simulink model "cwfd"  (R2019b)
settings: Solver=VariableStepAuto  StartTime=0.0  StopTime=10.0  RelTol=1e-3
settings Model: Creator=Blade  LastModifiedBy=Blade

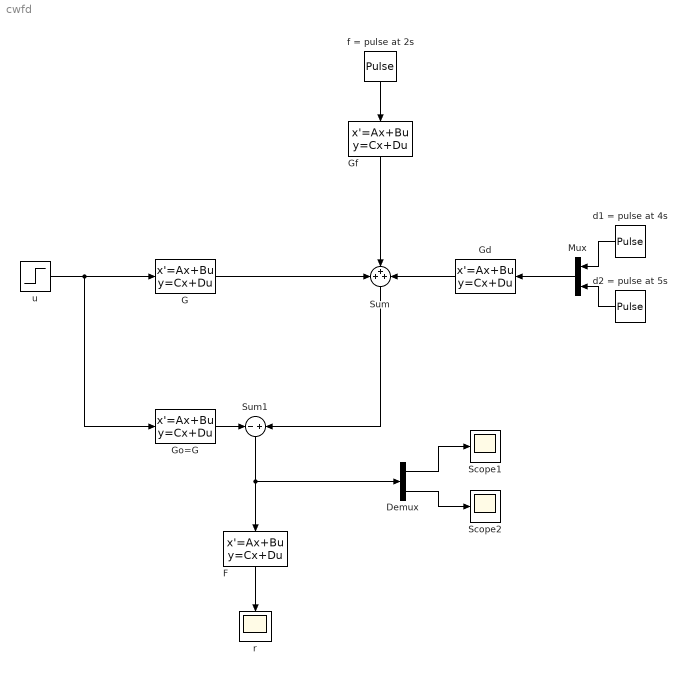
== system cwfd ==
  Demux : Demux  Outputs=2
  F : StateSpace  A=-26.6899  B=[60.7578,53.5442]  C=-0.1274  D=[0.1433,0.1401]  InitialCondition=0
  G : StateSpace  A=-2  C=[4;-5]  D=[0;0]  InitialCondition=0
  Gd : StateSpace  A=-2  B=[4,-4]  C=[4;-5]  D=[-4,0;3,2]  InitialCondition=0
  Gf : StateSpace  A=-2  C=[4;-5]  D=[6;1]  InitialCondition=0
  Go=G : StateSpace  A=-2  C=[4;-5]  D=[0;0]  InitialCondition=0
  Mux : Mux  Inputs=2
  "Scope1 " : Scope
  "Scope2 " : Scope
  Sum : Sum  Inputs=+++
  Sum1 : Sum  Inputs=-+
  d1 = pulse at 4s : DiscretePulseGenerator  PulseType=Time based  Amplitude=2  Period=10  PulseWidth=5  PhaseDelay=2
  d2 = pulse at 5s : DiscretePulseGenerator  PulseType=Time based  Amplitude=2  Period=10  PulseWidth=5  PhaseDelay=2
  f = pulse at 2s : DiscretePulseGenerator  PulseType=Time based  Amplitude=2  Period=10  PulseWidth=5  PhaseDelay=2
  r : Scope
  u : Step  SampleTime=0
  wires:
  f = pulse at 2s/1 -> Gf/1
  d1 = pulse at 4s/1 -> Mux/1
  d2 = pulse at 5s/1 -> Mux/2
  Mux/1 -> Gd/1
  G/1 -> Sum/1
  Gf/1 -> Sum/2
  Gd/1 -> Sum/3
  Go=G/1 -> Sum1/1
  Sum/1 -> Sum1/2
  Sum1/1 -> F/1, Demux/1
  F/1 -> r/1
  u/1 -> Go=G/1, G/1
  Demux/2 -> "Scope2 "/1
  Demux/1 -> "Scope1 "/1
